simulink model "Solar_Tracker_Model_Dual_axis"  (R2024a)
settings: Solver=ode45  StartTime=0.0  StopTime=24  MaxStep=0.01  RelTol=1e-3
PreLoadFcn:
  | addpath(fullfile('WormAndGearConstraintSupport','Data'));
  | addpath(fullfile('WormAndGearConstraintSupport','Scripts'));
model workspace: external: MATLAB File WormAndGearConstraintParameters.m (data not in the file)
undefined symbols (not defined in the file or in its folder): X, Y, Z
libraries: fl_lib x42, nesl_utility x18, WormAndGearConstraintLibrary x18, fl_ps_legacy_lib x17, sm_lib x9, ee_lib x4, simulink x2, SignalEditorBlockLib x2
(part 2 of 2)

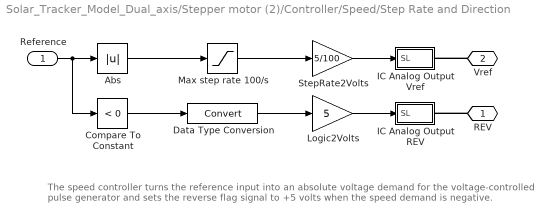
== system Solar_Tracker_Model_Dual_axis/Stepper motor (2)/Controller/Speed/Step Rate and Direction ==
  note: The speed controller turns the reference input into an absolute voltage demand for the
      | voltage-controlled pulse generator and sets the reverse flag signal to +5 volts when the
      | speed demand is negative.
  Reference : Inport
  Abs : Abs  SaturateOnIntegerOverflow=off
  Compare To Constant : simulink/Logic and Bit Operations/Compare To Constant  relop=<  const=0  OutDataTypeStr=uint8  ZeroCross=off
  Data Type Conversion : DataTypeConversion  SaturateOnIntegerOverflow=off  RndMeth=Floor
  IC Analog Output REV : Subsystem
  IC Analog Output Vref : Subsystem
  Logic2Volts : Gain  Gain=5
  Max step rate 100/s : Saturate  UpperLimit=100  LowerLimit=0
  StepRate2Volts : Gain  Gain=5/100
  REV : PMIOPort  Side=Right
  Vref : PMIOPort  Port=2  Side=Right
  wires:
  StepRate2Volts/1 -> IC Analog Output Vref/1(SL)
  Max step rate 100/s/1 -> StepRate2Volts/1
  Data Type Conversion/1 -> Logic2Volts/1
  Compare To Constant/1 -> Data Type Conversion/1
  Reference/1 -> Compare To Constant/1, Abs/1
  Abs/1 -> Max step rate 100/s/1
  Logic2Volts/1 -> IC Analog Output REV/1(SL)
  connections:
  REV/RConn1 -- IC Analog Output REV/RConn1
  Vref/RConn1 -- IC Analog Output Vref/RConn1

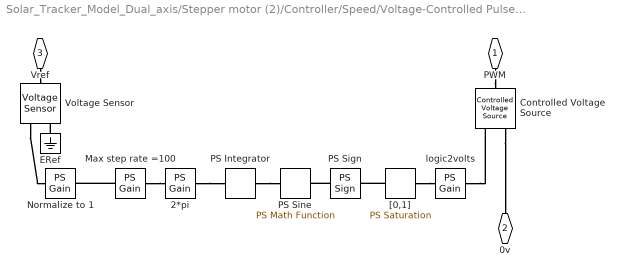
== system Solar_Tracker_Model_Dual_axis/Stepper motor (2)/Controller/Speed/Voltage-Controlled Pulse Generator ==
  2*pi : fl_ps_legacy_lib/Legacy Physical Signals/Functions/PS Gain  gain=-2*pi
  Controlled Voltage Source : fl_lib/Electrical/Electrical Sources/Controlled Voltage Source
  ERef : fl_lib/Electrical/Electrical Elements/Electrical Reference
  Max step rate =100 : fl_ps_legacy_lib/Legacy Physical Signals/Functions/PS Gain  gain=100
  Normalize to 1 : fl_ps_legacy_lib/Legacy Physical Signals/Functions/PS Gain  gain=1/5
  PS Integrator : fl_ps_legacy_lib/Legacy Physical Signals/Linear Operators/PS Integrator  x0=0
      settings: InternalSimscapePortConfiguration="{\"Bottom\":[],\"Left\":[{\"id\":\"I\",\"label\":\"\",\"type\":\"input\"}],\"Right\":[{\"id\":\"O\",\"label\":\"\",\"type\":\"output\"}],\"Top\":[]}"
  PS Sign : fl_ps_legacy_lib/Legacy Physical Signals/Nonlinear Operators/PS Sign
      settings: InternalSimscapePortConfiguration="{\"Bottom\":[],\"Left\":[{\"id\":\"I\",\"label\":\"\",\"type\":\"input\"}],\"Right\":[{\"id\":\"O\",\"label\":\"\",\"type\":\"output\"}],\"Top\":[]}"
  PS Sine : fl_ps_legacy_lib/Legacy Physical Signals/Functions/PS Math Function  fcn_choice=1
      settings: InternalSimscapePortConfiguration="{\"Bottom\":[],\"Left\":[{\"id\":\"I\",\"label\":\"\",\"type\":\"input\"}],\"Right\":[{\"id\":\"O\",\"label\":\"\",\"type\":\"output\"}],\"Top\":[]}"
  Voltage Sensor : fl_lib/Electrical/Electrical Sensors/Voltage Sensor
  "[0,1]" : fl_ps_legacy_lib/Legacy Physical Signals/Nonlinear Operators/PS Saturation  upper_limit=1  lower_limit=0
      settings: InternalSimscapePortConfiguration="{\"Bottom\":[],\"Left\":[{\"id\":\"I\",\"label\":\"\",\"type\":\"input\"}],\"Right\":[{\"id\":\"O\",\"label\":\"\",\"type\":\"output\"}],\"Top\":[]}"
  logic2volts : fl_ps_legacy_lib/Legacy Physical Signals/Functions/PS Gain  gain=5
  PWM : PMIOPort  Side=Right
  0v : PMIOPort  Port=2  Side=Right
  Vref : PMIOPort  Port=3  Side=Left
  connections:
  PWM/RConn1 -- Controlled Voltage Source/LConn1
  Controlled Voltage Source/RConn2 -- 0v/RConn1
  Vref/RConn1 -- Voltage Sensor/LConn1
  ERef/LConn1 -- Voltage Sensor/RConn2
  Voltage Sensor/RConn1 -- Normalize to 1/LConn1
  Max step rate =100/LConn1 -- Normalize to 1/RConn1
  Max step rate =100/RConn1 -- 2*pi/LConn1
  2*pi/RConn1 -- PS Integrator/LConn1
  PS Integrator/RConn1 -- PS Sine/LConn1
  PS Sign/LConn1 -- PS Sine/RConn1
  "[0,1]"/LConn1 -- PS Sign/RConn1
  "[0,1]"/RConn1 -- logic2volts/LConn1
  logic2volts/RConn1 -- Controlled Voltage Source/RConn1

== system Solar_Tracker_Model_Dual_axis/Subsystem/Solar Array/Solar Tracker1/Solar Panel Assembly ==
  Frame : WormAndGearConstraintLibrary/Frame  width=frame.width  height=frame.height  depth=frame.depth  beamWidth=frame.beamWidth  beamThickness=frame.beamThickness  frameWidth=frame.frameWidth  frameThickness=frame.frameThickness  rho=frame.density  beamColor=frame.beamColor  frameColor=frame.frameColor
      settings: LibrarySourceBlock=sm_solar_tracker_lib/Frame
  Frame Mount : WormAndGearConstraintLibrary/Frame Mount  bracketWidth=framemount.bracketWidthHeight  bracketThickness=framemount.bracketThickness  bracketOffset=framemount.bracketOffset  holeRadius=framemount.holeRadius  holeOffset=framemount.holeOffset  baseThickness=framemount.baseThickness  rho=framemount.density  mountColor=framemount.mountColor  pinColor=framemount.pinColor
      settings: LibrarySourceBlock=sm_solar_tracker_lib/Frame Mount
  Solar Panel : WormAndGearConstraintLibrary/Solar Panel  width=solarpanel.width  height=solarpanel.height  frameWidth=solarpanel.frameWidth  frameDepth=solarpanel.frameDepth  cellsRho=solarpanel.cellDensity  frameRho=solarpanel.frameDensity  cellsColor=solarpanel.cellColor  frameColor=solarpanel.frameColor
      settings: LibrarySourceBlock=sm_solar_tracker_lib/Solar Panel
  H : PMIOPort  Side=Left
  connections:
  Frame/RConn1 -- Solar Panel/LConn1
  Frame Mount/LConn1 -- Frame/LConn1
  H/RConn1 -- Frame Mount/RConn1

== system Solar_Tracker_Model_Dual_axis/Subsystem/Solar Array/Solar Tracker2/Solar Panel Assembly ==
  Frame : WormAndGearConstraintLibrary/Frame  width=frame.width  height=frame.height  depth=frame.depth  beamWidth=frame.beamWidth  beamThickness=frame.beamThickness  frameWidth=frame.frameWidth  frameThickness=frame.frameThickness  rho=frame.density  beamColor=frame.beamColor  frameColor=frame.frameColor
      settings: LibrarySourceBlock=sm_solar_tracker_lib/Frame
  Frame Mount : WormAndGearConstraintLibrary/Frame Mount  bracketWidth=framemount.bracketWidthHeight  bracketThickness=framemount.bracketThickness  bracketOffset=framemount.bracketOffset  holeRadius=framemount.holeRadius  holeOffset=framemount.holeOffset  baseThickness=framemount.baseThickness  rho=framemount.density  mountColor=framemount.mountColor  pinColor=framemount.pinColor
      settings: LibrarySourceBlock=sm_solar_tracker_lib/Frame Mount
  Solar Panel : WormAndGearConstraintLibrary/Solar Panel  width=solarpanel.width  height=solarpanel.height  frameWidth=solarpanel.frameWidth  frameDepth=solarpanel.frameDepth  cellsRho=solarpanel.cellDensity  frameRho=solarpanel.frameDensity  cellsColor=solarpanel.cellColor  frameColor=solarpanel.frameColor
      settings: LibrarySourceBlock=sm_solar_tracker_lib/Solar Panel
  H : PMIOPort  Side=Left
  connections:
  H/RConn1 -- Frame Mount/RConn1
  Frame Mount/LConn1 -- Frame/LConn1
  Frame/RConn1 -- Solar Panel/LConn1

== system Solar_Tracker_Model_Dual_axis/Subsystem/Solar Array/Solar Tracker3/Solar Panel Assembly ==
  Frame : WormAndGearConstraintLibrary/Frame  width=frame.width  height=frame.height  depth=frame.depth  beamWidth=frame.beamWidth  beamThickness=frame.beamThickness  frameWidth=frame.frameWidth  frameThickness=frame.frameThickness  rho=frame.density  beamColor=frame.beamColor  frameColor=frame.frameColor
      settings: LibrarySourceBlock=sm_solar_tracker_lib/Frame
  Frame Mount : WormAndGearConstraintLibrary/Frame Mount  bracketWidth=framemount.bracketWidthHeight  bracketThickness=framemount.bracketThickness  bracketOffset=framemount.bracketOffset  holeRadius=framemount.holeRadius  holeOffset=framemount.holeOffset  baseThickness=framemount.baseThickness  rho=framemount.density  mountColor=framemount.mountColor  pinColor=framemount.pinColor
      settings: LibrarySourceBlock=sm_solar_tracker_lib/Frame Mount
  Solar Panel : WormAndGearConstraintLibrary/Solar Panel  width=solarpanel.width  height=solarpanel.height  frameWidth=solarpanel.frameWidth  frameDepth=solarpanel.frameDepth  cellsRho=solarpanel.cellDensity  frameRho=solarpanel.frameDensity  cellsColor=solarpanel.cellColor  frameColor=solarpanel.frameColor
      settings: LibrarySourceBlock=sm_solar_tracker_lib/Solar Panel
  H : PMIOPort  Side=Left
  connections:
  Frame/RConn1 -- Solar Panel/LConn1
  Frame Mount/LConn1 -- Frame/LConn1
  H/RConn1 -- Frame Mount/RConn1

== system Solar_Tracker_Model_Dual_axis/Stepper motor (1)/Controller1/Position/Algorithm and Pulse Generation/IC Analog Output REV ==
  SL : Inport
  Controlled Voltage Source : fl_lib/Electrical/Electrical Sources/Controlled Voltage Source
  ERef : fl_lib/Electrical/Electrical Elements/Electrical Reference
  Simulink-PS Converter : nesl_utility/Simulink-PS Converter  PhysicalDomain=network_engine_domain  SubClassName=ps_input  LeftPortType=input  RightPortType=output  PseudoPeriodic=off  Frequencies=[]  NoiseDistribution=none  NoiseParameters=[]  Unit=V  AffineConversion=off  FilteringAndDerivatives=zero  SimscapeFilterOrder=1  InputFilterTimeConstant=.001  UdotUserProvided=0
  V : PMIOPort  Side=Right
  wires:
  SL/1 -> Simulink-PS Converter/1
  connections:
  ERef/LConn1 -- Controlled Voltage Source/RConn2
  V/RConn1 -- Controlled Voltage Source/LConn1
  Simulink-PS Converter/RConn1 -- Controlled Voltage Source/RConn1

== system Solar_Tracker_Model_Dual_axis/Stepper motor (1)/Controller1/Position/Algorithm and Pulse Generation/IC Analog Output Vref ==
  SL : Inport
  Controlled Voltage Source : fl_lib/Electrical/Electrical Sources/Controlled Voltage Source
  ERef : fl_lib/Electrical/Electrical Elements/Electrical Reference
  Simulink-PS Converter : nesl_utility/Simulink-PS Converter  PhysicalDomain=network_engine_domain  SubClassName=ps_input  LeftPortType=input  RightPortType=output  PseudoPeriodic=off  Frequencies=[]  NoiseDistribution=none  NoiseParameters=[]  Unit=V  AffineConversion=off  FilteringAndDerivatives=zero  SimscapeFilterOrder=1  InputFilterTimeConstant=.001  UdotUserProvided=0
  V : PMIOPort  Side=Right
  wires:
  SL/1 -> Simulink-PS Converter/1
  connections:
  Simulink-PS Converter/RConn1 -- Controlled Voltage Source/RConn1
  V/RConn1 -- Controlled Voltage Source/LConn1
  ERef/LConn1 -- Controlled Voltage Source/RConn2

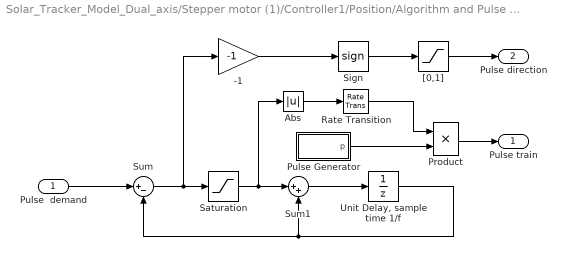
== system Solar_Tracker_Model_Dual_axis/Stepper motor (1)/Controller1/Position/Algorithm and Pulse Generation/Pulse Generator ==
  Pulse  demand : Inport  SampleTime=1/f
  -1 : Gain  Gain=-1
  Abs : Abs  SaturateOnIntegerOverflow=off
  Product : Product  InputSameDT=on  SaturateOnIntegerOverflow=on  OutDataTypeStr=Inherit: Same as first input
  Pulse Generator : Subsystem
  Rate Transition : RateTransition  Deterministic=off
  Saturation : Saturate  UpperLimit=1  LowerLimit=-1
  Sign : Signum
  Sum : Sum  Inputs=|+-
  Sum1 : Sum  Inputs=|++
  "Unit Delay, sample time 1/f" : UnitDelay  SampleTime=1/f  HasFrameUpgradeWarning=on
  "[0,1]" : Saturate  UpperLimit=1  LowerLimit=0
  Pulse train : Outport  VectorParamsAs1DForOutWhenUnconnected=off
  Pulse direction : Outport  Port=2  VectorParamsAs1DForOutWhenUnconnected=off
  wires:
  "[0,1]"/1 -> Pulse direction/1
  -1/1 -> Sign/1
  "Unit Delay, sample time 1/f"/1 -> Sum/2, Sum1/2
  Pulse  demand/1 -> Sum/1
  Sum/1 -> -1/1, Saturation/1
  Saturation/1 -> Sum1/1, Abs/1
  Sum1/1 -> "Unit Delay, sample time 1/f"/1
  Sign/1 -> "[0,1]"/1
  Product/1 -> Pulse train/1
  Abs/1 -> Rate Transition/1
  Pulse Generator/1(p) -> Product/2
  Rate Transition/1 -> Product/1

== system Solar_Tracker_Model_Dual_axis/Stepper motor (1)/Controller1/Speed/Step Rate and Direction/IC Analog Output REV ==
  SL : Inport
  Controlled Voltage Source : fl_lib/Electrical/Electrical Sources/Controlled Voltage Source
  ERef : fl_lib/Electrical/Electrical Elements/Electrical Reference
  Simulink-PS Converter : nesl_utility/Simulink-PS Converter  PhysicalDomain=network_engine_domain  SubClassName=ps_input  LeftPortType=input  RightPortType=output  PseudoPeriodic=off  Frequencies=[]  NoiseDistribution=none  NoiseParameters=[]  Unit=V  AffineConversion=off  FilteringAndDerivatives=zero  SimscapeFilterOrder=1  InputFilterTimeConstant=.001  UdotUserProvided=0
  V : PMIOPort  Side=Right
  wires:
  SL/1 -> Simulink-PS Converter/1
  connections:
  Simulink-PS Converter/RConn1 -- Controlled Voltage Source/RConn1
  V/RConn1 -- Controlled Voltage Source/LConn1
  ERef/LConn1 -- Controlled Voltage Source/RConn2

== system Solar_Tracker_Model_Dual_axis/Stepper motor (1)/Controller1/Speed/Step Rate and Direction/IC Analog Output Vref ==
  SL : Inport
  Controlled Voltage Source : fl_lib/Electrical/Electrical Sources/Controlled Voltage Source
  ERef : fl_lib/Electrical/Electrical Elements/Electrical Reference
  Simulink-PS Converter : nesl_utility/Simulink-PS Converter  PhysicalDomain=network_engine_domain  SubClassName=ps_input  LeftPortType=input  RightPortType=output  PseudoPeriodic=off  Frequencies=[]  NoiseDistribution=none  NoiseParameters=[]  Unit=V  AffineConversion=off  FilteringAndDerivatives=zero  SimscapeFilterOrder=1  InputFilterTimeConstant=.001  UdotUserProvided=0
  V : PMIOPort  Side=Right
  wires:
  SL/1 -> Simulink-PS Converter/1
  connections:
  ERef/LConn1 -- Controlled Voltage Source/RConn2
  V/RConn1 -- Controlled Voltage Source/LConn1
  Simulink-PS Converter/RConn1 -- Controlled Voltage Source/RConn1

== system Solar_Tracker_Model_Dual_axis/Stepper motor (2)/Controller/Position/Algorithm and Pulse Generation/IC Analog Output REV ==
  SL : Inport
  Controlled Voltage Source : fl_lib/Electrical/Electrical Sources/Controlled Voltage Source
  ERef : fl_lib/Electrical/Electrical Elements/Electrical Reference
  Simulink-PS Converter : nesl_utility/Simulink-PS Converter  PhysicalDomain=network_engine_domain  SubClassName=ps_input  LeftPortType=input  RightPortType=output  PseudoPeriodic=off  Frequencies=[]  NoiseDistribution=none  NoiseParameters=[]  Unit=V  AffineConversion=off  FilteringAndDerivatives=zero  SimscapeFilterOrder=1  InputFilterTimeConstant=.001  UdotUserProvided=0
  V : PMIOPort  Side=Right
  wires:
  SL/1 -> Simulink-PS Converter/1
  connections:
  ERef/LConn1 -- Controlled Voltage Source/RConn2
  V/RConn1 -- Controlled Voltage Source/LConn1
  Simulink-PS Converter/RConn1 -- Controlled Voltage Source/RConn1

== system Solar_Tracker_Model_Dual_axis/Stepper motor (2)/Controller/Position/Algorithm and Pulse Generation/IC Analog Output Vref ==
  SL : Inport
  Controlled Voltage Source : fl_lib/Electrical/Electrical Sources/Controlled Voltage Source
  ERef : fl_lib/Electrical/Electrical Elements/Electrical Reference
  Simulink-PS Converter : nesl_utility/Simulink-PS Converter  PhysicalDomain=network_engine_domain  SubClassName=ps_input  LeftPortType=input  RightPortType=output  PseudoPeriodic=off  Frequencies=[]  NoiseDistribution=none  NoiseParameters=[]  Unit=V  AffineConversion=off  FilteringAndDerivatives=zero  SimscapeFilterOrder=1  InputFilterTimeConstant=.001  UdotUserProvided=0
  V : PMIOPort  Side=Right
  wires:
  SL/1 -> Simulink-PS Converter/1
  connections:
  Simulink-PS Converter/RConn1 -- Controlled Voltage Source/RConn1
  V/RConn1 -- Controlled Voltage Source/LConn1
  ERef/LConn1 -- Controlled Voltage Source/RConn2

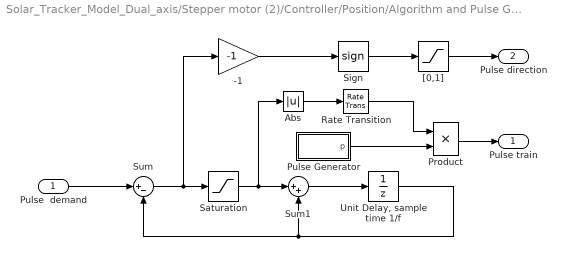
== system Solar_Tracker_Model_Dual_axis/Stepper motor (2)/Controller/Position/Algorithm and Pulse Generation/Pulse Generator ==
  Pulse  demand : Inport  SampleTime=1/f
  -1 : Gain  Gain=-1
  Abs : Abs  SaturateOnIntegerOverflow=off
  Product : Product  InputSameDT=on  SaturateOnIntegerOverflow=on  OutDataTypeStr=Inherit: Same as first input
  Pulse Generator : Subsystem
  Rate Transition : RateTransition  Deterministic=off
  Saturation : Saturate  UpperLimit=1  LowerLimit=-1
  Sign : Signum
  Sum : Sum  Inputs=|+-
  Sum1 : Sum  Inputs=|++
  "Unit Delay, sample time 1/f" : UnitDelay  SampleTime=1/f  HasFrameUpgradeWarning=on
  "[0,1]" : Saturate  UpperLimit=1  LowerLimit=0
  Pulse train : Outport  VectorParamsAs1DForOutWhenUnconnected=off
  Pulse direction : Outport  Port=2  VectorParamsAs1DForOutWhenUnconnected=off
  wires:
  "[0,1]"/1 -> Pulse direction/1
  -1/1 -> Sign/1
  "Unit Delay, sample time 1/f"/1 -> Sum/2, Sum1/2
  Pulse  demand/1 -> Sum/1
  Sum/1 -> -1/1, Saturation/1
  Saturation/1 -> Sum1/1, Abs/1
  Sum1/1 -> "Unit Delay, sample time 1/f"/1
  Sign/1 -> "[0,1]"/1
  Product/1 -> Pulse train/1
  Abs/1 -> Rate Transition/1
  Pulse Generator/1(p) -> Product/2
  Rate Transition/1 -> Product/1

== system Solar_Tracker_Model_Dual_axis/Stepper motor (2)/Controller/Speed/Step Rate and Direction/IC Analog Output REV ==
  SL : Inport
  Controlled Voltage Source : fl_lib/Electrical/Electrical Sources/Controlled Voltage Source
  ERef : fl_lib/Electrical/Electrical Elements/Electrical Reference
  Simulink-PS Converter : nesl_utility/Simulink-PS Converter  PhysicalDomain=network_engine_domain  SubClassName=ps_input  LeftPortType=input  RightPortType=output  PseudoPeriodic=off  Frequencies=[]  NoiseDistribution=none  NoiseParameters=[]  Unit=V  AffineConversion=off  FilteringAndDerivatives=zero  SimscapeFilterOrder=1  InputFilterTimeConstant=.001  UdotUserProvided=0
  V : PMIOPort  Side=Right
  wires:
  SL/1 -> Simulink-PS Converter/1
  connections:
  Simulink-PS Converter/RConn1 -- Controlled Voltage Source/RConn1
  V/RConn1 -- Controlled Voltage Source/LConn1
  ERef/LConn1 -- Controlled Voltage Source/RConn2

== system Solar_Tracker_Model_Dual_axis/Stepper motor (2)/Controller/Speed/Step Rate and Direction/IC Analog Output Vref ==
  SL : Inport
  Controlled Voltage Source : fl_lib/Electrical/Electrical Sources/Controlled Voltage Source
  ERef : fl_lib/Electrical/Electrical Elements/Electrical Reference
  Simulink-PS Converter : nesl_utility/Simulink-PS Converter  PhysicalDomain=network_engine_domain  SubClassName=ps_input  LeftPortType=input  RightPortType=output  PseudoPeriodic=off  Frequencies=[]  NoiseDistribution=none  NoiseParameters=[]  Unit=V  AffineConversion=off  FilteringAndDerivatives=zero  SimscapeFilterOrder=1  InputFilterTimeConstant=.001  UdotUserProvided=0
  V : PMIOPort  Side=Right
  wires:
  SL/1 -> Simulink-PS Converter/1
  connections:
  ERef/LConn1 -- Controlled Voltage Source/RConn2
  V/RConn1 -- Controlled Voltage Source/LConn1
  Simulink-PS Converter/RConn1 -- Controlled Voltage Source/RConn1

== system Solar_Tracker_Model_Dual_axis/Stepper motor (1)/Controller1/Position/Algorithm and Pulse Generation/Pulse Generator/Pulse Generator ==
  -1 : Gain  Gain=0.5
  Constant : Constant  SampleTime=1/(2*f)
  Gain : Gain  Gain=-1
  Sum : Sum  Inputs=|++
  "Unit Delay, sample time 1/2*f)" : UnitDelay  InitialCondition=-1  SampleTime=1/(2*f)  HasFrameUpgradeWarning=on
  p : Outport  VectorParamsAs1DForOutWhenUnconnected=off
  wires:
  "Unit Delay, sample time 1/2*f)"/1 -> Gain/1, Sum/1
  Gain/1 -> "Unit Delay, sample time 1/2*f)"/1
  Constant/1 -> Sum/2
  Sum/1 -> -1/1
  -1/1 -> p/1

== system Solar_Tracker_Model_Dual_axis/Stepper motor (2)/Controller/Position/Algorithm and Pulse Generation/Pulse Generator/Pulse Generator ==
  -1 : Gain  Gain=0.5
  Constant : Constant  SampleTime=1/(2*f)
  Gain : Gain  Gain=-1
  Sum : Sum  Inputs=|++
  "Unit Delay, sample time 1/2*f)" : UnitDelay  InitialCondition=-1  SampleTime=1/(2*f)  HasFrameUpgradeWarning=on
  p : Outport  VectorParamsAs1DForOutWhenUnconnected=off
  wires:
  "Unit Delay, sample time 1/2*f)"/1 -> Gain/1, Sum/1
  Gain/1 -> "Unit Delay, sample time 1/2*f)"/1
  Constant/1 -> Sum/2
  Sum/1 -> -1/1
  -1/1 -> p/1
